simulink model "quadcopter_process_test"  (R2015b)
settings: Solver=VariableStepAuto  StartTime=0.0  StopTime=2  RelTol=1e-3
libraries: vrlib x2
settings Model: Creator=Daniel  LastModifiedBy=mgreiff

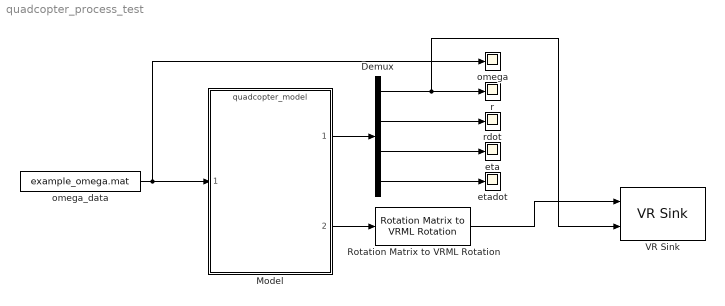
== system quadcopter_process_test ==
  Demux : Demux  Outputs=[3,3,3,3]
  Model : ModelReference  ModelNameDialog=quadcopter_model.mdl  SimulationMode=Normal  ModelReferenceVersion=1.117  CopyOfModelName=quadcopter_model.mdl
  Rotation Matrix to VRML Rotation : vrlib/Utilities/Rotation Matrix to VRML Rotation  maxzero=1e-12
  VR Sink : vrlib/VR Sink  InstantiateOnLoad=on  SampleTime=0.1  ViewEnable=on  RemoteChange=off  RemoteView=off  FieldsWritten=copter.rotation.4.1.1.double#copter.translation.3.1.1.double  WorldFileName=copter_world.wrl  AutoView=on  VideoDimensions=[]  AllowVariableSize=off
  eta : Scope
  etadot : Scope
  omega : Scope
  omega_data : FromFile  FileName=example_omega.mat  SampleTime=0.01
  r : Scope
  rdot : Scope
  wires:
  omega_data/1 -> omega/1, Model/1
  Rotation Matrix to VRML Rotation/1 -> VR Sink/1
  Model/2 -> Rotation Matrix to VRML Rotation/1
  Model/1 -> Demux/1
  Demux/3 -> eta/1
  Demux/2 -> rdot/1
  Demux/1 -> VR Sink/2, r/1
  Demux/4 -> etadot/1
